simulink model "QRotorSimulation_previousversion2020"  (R2019a)
settings: Solver=FixedStepAuto  StartTime=0.0  StopTime=100  FixedStep=0.001  RelTol=1e-9
values from neighbouring files (symbols this model uses):
  K = lqr(A, B, Q, R)    [Linear_model.m]    (also in project_disturbance_observer.m = lqr(A_LD,B_LD,Q,R))
libraries: simulink x1
settings Model: Creator=carlossilvestre  LastModifiedBy=yulinchen

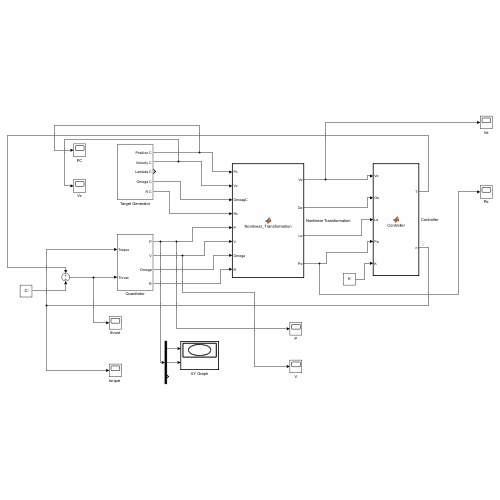
[thumbnail: Simulink's stored preview of the top-level diagram]
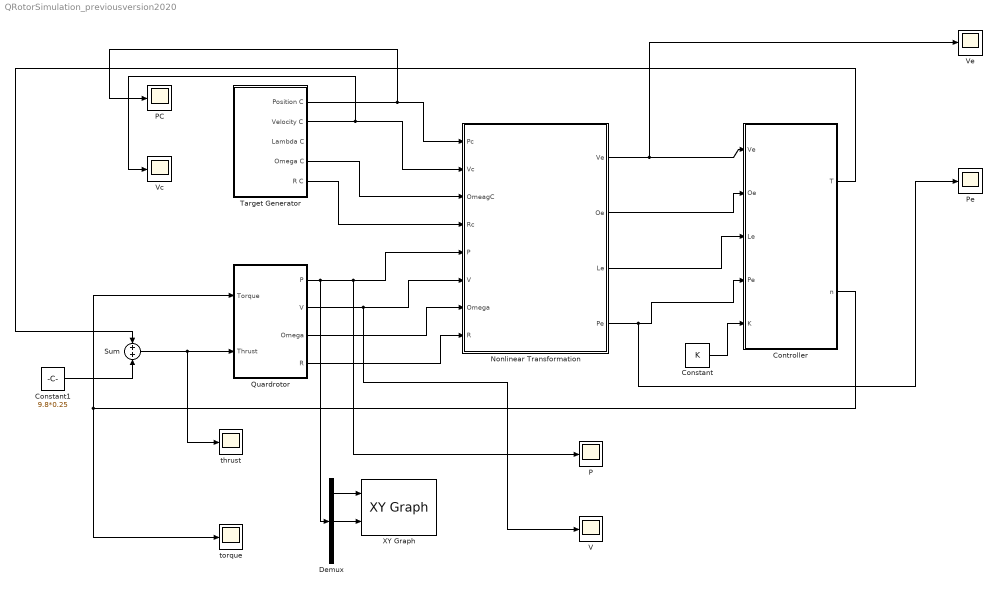
== system QRotorSimulation_previousversion2020 ==
  Constant : Constant  Value=K
  Constant1 : Constant  Value=9.8*0.25
  Controller : MATLAB Function  TreatAsAtomicUnit=on
  Demux : Demux  Outputs=3
  Nonlinear Transformation : MATLAB Function  TreatAsAtomicUnit=on
  P : Scope
  PC : Scope
  Pe : Scope
  Quardrotor : Subsystem
  Sum : Sum
  Target Generator : Subsystem
  V : Scope
  Vc : Scope
  Ve : Scope
  XY Graph : simulink/Sinks/XY Graph  xmin=-1  xmax=1  ymin=-1  ymax=1  st=-1
  thrust : Scope
  "torque " : Scope
  wires:
  Target Generator/1(Position C) -> PC/1, Nonlinear Transformation/1(Pc)
  Target Generator/2(Velocity C) -> Vc/1, Nonlinear Transformation/2(Vc)
  Target Generator/5(R C) -> Nonlinear Transformation/4(Rc)
  Quardrotor/1(P) -> P/1, Nonlinear Transformation/5(P), Demux/1
  Quardrotor/4(R) -> Nonlinear Transformation/8(R)
  Quardrotor/2(V) -> V/1, Nonlinear Transformation/6(V)
  Quardrotor/3(Omega) -> Nonlinear Transformation/7(Omega)
  Target Generator/4(Omega C) -> Nonlinear Transformation/3(OmeagC)
  Nonlinear Transformation/1(Ve) -> Ve/1, Controller/1(Ve)
  Nonlinear Transformation/2(Oe) -> Controller/2(Oe)
  Nonlinear Transformation/3(Le) -> Controller/3(Le)
  Nonlinear Transformation/4(Pe) -> Pe/1, Controller/4(Pe)
  Constant/1 -> Controller/5(K)
  Controller/1(T) -> Sum/1
  Controller/2(n) -> Quardrotor/1(Torque), "torque "/1
  Demux/1 -> XY Graph/1
  Demux/2 -> XY Graph/2
  Sum/1 -> thrust/1, Quardrotor/2(Thrust)
  Constant1/1 -> Sum/2

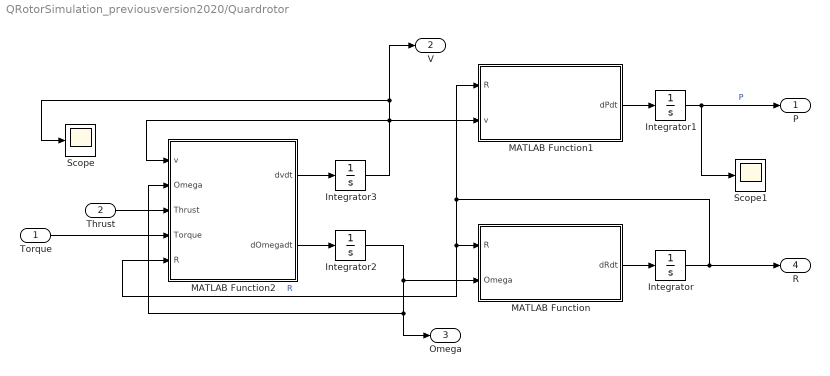
== system QRotorSimulation_previousversion2020/Quardrotor ==
  Torque : Inport
  Thrust : Inport  Port=2  PortDimensions=1
  Integrator : Integrator  InitialCondition=eye(3)
  Integrator1 : Integrator  InitialCondition=[0,0,0]
  Integrator2 : Integrator  InitialCondition=[0,0,0]  ContinuousStateAttributes='omega'
  Integrator3 : Integrator  InitialCondition=[0,0,0]  ContinuousStateAttributes='velocity'
  MATLAB Function : MATLAB Function  TreatAsAtomicUnit=on
  MATLAB Function1 : MATLAB Function  TreatAsAtomicUnit=on
  MATLAB Function2 : MATLAB Function  TreatAsAtomicUnit=on
  Scope : Scope
  Scope1 : Scope
  P : Outport
  V : Outport  Port=2
  Omega : Outport  Port=3
  R : Outport  Port=4
  wires:
  MATLAB Function2/1(dvdt) -> Integrator3/1
  Integrator1/1 -> Scope1/1, P/1  "P"
  Integrator2/1 -> MATLAB Function2/2(Omega), Omega/1, MATLAB Function/2(Omega)
  MATLAB Function/1(dRdt) -> Integrator/1
  MATLAB Function2/2(dOmegadt) -> Integrator2/1
  Integrator3/1 -> Scope/1, V/1, MATLAB Function2/1(v), MATLAB Function1/2(v)
  MATLAB Function1/1(dPdt) -> Integrator1/1
  Integrator/1 -> R/1, MATLAB Function1/1(R), MATLAB Function2/5(R), MATLAB Function/1(R)  "R"
  Thrust/1 -> MATLAB Function2/3(Thrust)
  Torque/1 -> MATLAB Function2/4(Torque)

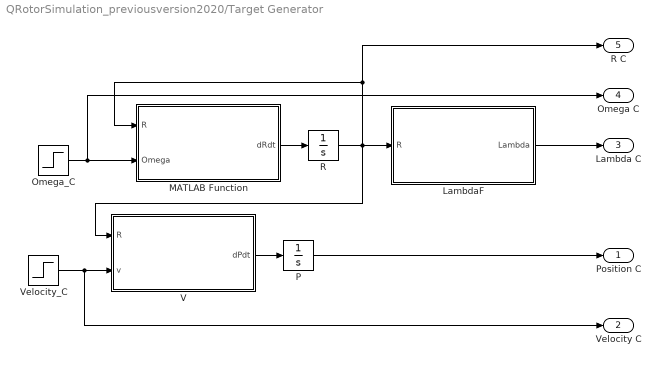
== system QRotorSimulation_previousversion2020/Target Generator ==
  LambdaF : MATLAB Function  TreatAsAtomicUnit=on
  MATLAB Function : MATLAB Function  TreatAsAtomicUnit=on
  Omega_C : Step  Time=0  Before=[0;0;0]  After=[0;0;0]  SampleTime=0
  P : Integrator
  R : Integrator  InitialCondition=eye(3)
  V : MATLAB Function  TreatAsAtomicUnit=on
  Velocity_C : Step  Time=0  Before=[1;2;0]  After=[1;2;0]  SampleTime=0
  Position C : Outport
  Velocity C : Outport  Port=2
  Lambda C : Outport  Port=3
  Omega C : Outport  Port=4
  R C : Outport  Port=5
  wires:
  LambdaF/1(Lambda) -> Lambda C/1
  P/1 -> Position C/1
  MATLAB Function/1(dRdt) -> R/1
  R/1 -> MATLAB Function/1(R), R C/1, V/1(R), LambdaF/1(R)
  V/1(dPdt) -> P/1
  Velocity_C/1 -> Velocity C/1, V/2(v)
  Omega_C/1 -> Omega C/1, MATLAB Function/2(Omega)

== matlab function QRotorSimulation_previousversion2020/Quardrotor/MATLAB Function1 ==
  data: R input; dPdt output; v input
function dPdt = CompdPdt(R,v)
dPdt=R*v;
end

== matlab function QRotorSimulation_previousversion2020/Quardrotor/MATLAB Function ==
  data: R input; dRdt output; Omega input
function dRdt = CompdRdt(R,Omega)
dRdt=R*skew(Omega);
end

== matlab function QRotorSimulation_previousversion2020/Quardrotor/MATLAB Function2 ==
  data: v input; Omega input; dvdt output; Thrust input; Torque input; dOmegadt output; R input
function [dvdt,dOmegadt] = Dynamics(v,Omega,Thrust,Torque,R)

m = 0.25;
g = 9.8;
I = 0.1 * eye(3);

dvdt = -skew(Omega)*v - 1/m * Thrust * [0;0;1] + R' * [0;0;g] ;
dOmegadt = -I^-1 * skew(Omega) * I * Omega + I^-1 * Torque ;

end

== matlab function QRotorSimulation_previousversion2020/Target Generator/V ==
  data: R input; dPdt output; v input
function dPdt = CompdPdt(R,v)
dPdt=R*v;
end

== matlab function QRotorSimulation_previousversion2020/Controller ==
  data: Ve input; Oe input; Le input; Pe input; T output; n output; K input
function [T,n] = Controller(Ve,Oe,Le,Pe,K)

State = [Pe; Ve; Le; Oe];
Cntl = -K * State;
T = Cntl(1);
n = Cntl(2:4);


end

== matlab function QRotorSimulation_previousversion2020/Nonlinear Transformation ==
  data: Pc input; Vc input; OmeagC input; Rc input; P input; V input; Omega input; R input; Ve output; Oe output; Le output; Pe output
function [Ve,Oe,Le,Pe] = Nonlinear_Transformation(Pc,Vc,OmeagC,Rc,P,V,Omega,R)

Ve = V - Vc;
Oe = Omega - OmeagC;
Pe = P - Pc;
Re = R * Rc';

Pitch = atan2(-Re(3,1),sqrt(Re(1,1)^2 + Re(2,1)^2));
Yaw = atan2(Re(2,1)/cos(Pitch),Re(1,1)/cos(Pitch));
Roll = atan2(Re(3,2)/cos(Pitch),Re(3,3)/cos(Pitch));
Le = [Roll;Pitch;Yaw];

end

== matlab function QRotorSimulation_previousversion2020/Target Generator/LambdaF ==
  data: R input; Lambda output
function Lambda = R_to_Lambda(R)

Pitch = atan2(-R(3,1),sqrt(R(1,1)^2 + R(2,1)^2));
Yaw = atan2(R(2,1)/cos(Pitch),R(1,1)/cos(Pitch));
Roll = atan2(R(3,2)/cos(Pitch),R(3,3)/cos(Pitch));
Lambda = [Roll;Pitch;Yaw];

end

== matlab function QRotorSimulation_previousversion2020/Target Generator/MATLAB Function ==
  data: R input; dRdt output; Omega input
function dRdt = CompdRdt(R,Omega)
dRdt=R*skew(Omega);
end
